simulink model "modelo_i"  (R2026a)
settings: Solver=VariableStepAuto  StopTime=1000  FixedStep=1
values from neighbouring files (symbols this model uses):
  theta = 5    [init.m]
settings Model: Creator=honda  LastModifiedBy=honda

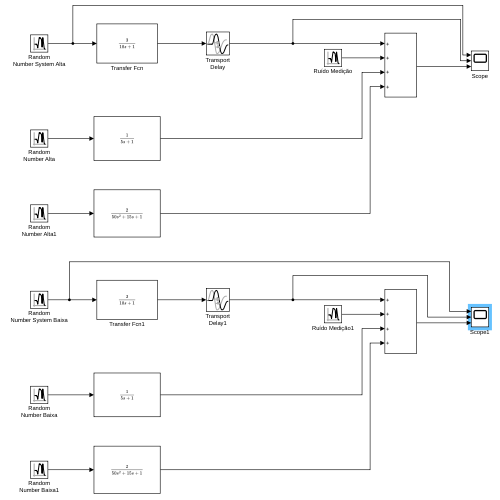
[thumbnail: Simulink's stored preview of the top-level diagram]
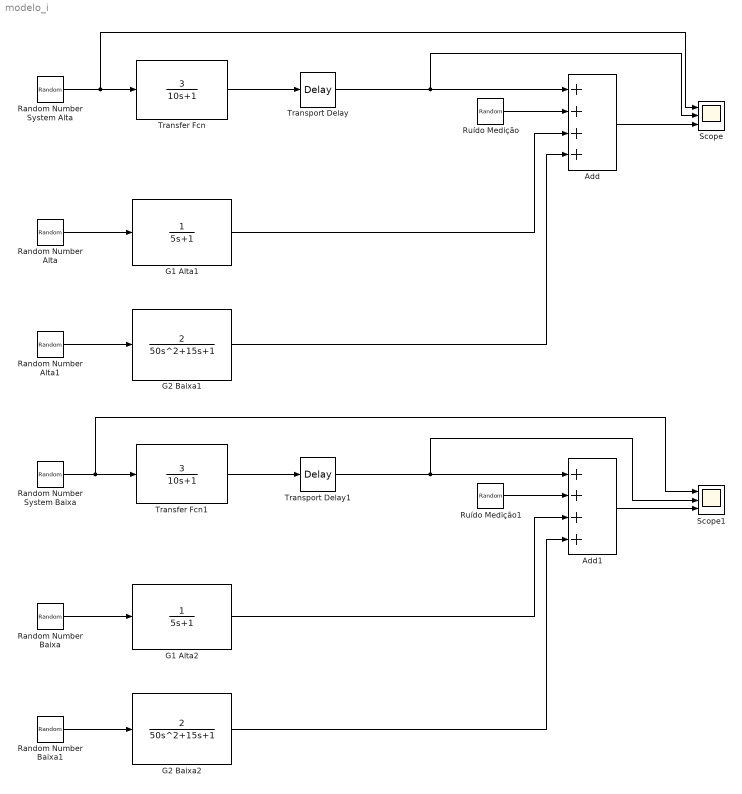
== system modelo_i ==
  Add : Sum  Inputs=++++
  Add1 : Sum  Inputs=++++
  G1 Alta1 : TransferFcn  Denominator=[5 1]
  G1 Alta2 : TransferFcn  Denominator=[5 1]
  G2 Baixa1 : TransferFcn  Numerator=[2]  Denominator=[50 15 1]
  G2 Baixa2 : TransferFcn  Numerator=[2]  Denominator=[50 15 1]
  Random Number Alta : RandomNumber  Variance=0.1  Seed=123  SampleTime=1
  Random Number Alta1 : RandomNumber  Variance=0.1  Seed=456  SampleTime=1
  Random Number Baixa : RandomNumber  Variance=0.001  SampleTime=1
  Random Number Baixa1 : RandomNumber  Variance=0.001  SampleTime=1
  Random Number System Alta : RandomNumber  Variance=0.1  Seed=100  SampleTime=1
  Random Number System Baixa : RandomNumber  Variance=0.1  Seed=100  SampleTime=1
  Ruído Medição : RandomNumber  Variance=1e-6  SampleTime=0.01
  Ruído Medição1 : RandomNumber  Variance=1e-6  SampleTime=0.01
  Scope : Scope  NumInputPorts=3
      settings: ActiveDisplayYMinimum=-1  ActiveDisplayYMaximum=1  DataLoggingVariableName=dados_i_alta
  Scope1 : Scope  NumInputPorts=3
      settings: ActiveDisplayYMinimum=-1  ActiveDisplayYMaximum=1  DataLoggingVariableName=dados_i_baixa
  Transfer Fcn : TransferFcn  Numerator=[3]  Denominator=[10 1]
  Transfer Fcn1 : TransferFcn  Numerator=[3]  Denominator=[10 1]
  Transport Delay : TransportDelay  DelayTime=theta
  Transport Delay1 : TransportDelay  DelayTime=theta
  wires:
  Random Number System Alta/1 -> Scope/1, Transfer Fcn/1
  Transfer Fcn/1 -> Transport Delay/1
  Random Number Alta/1 -> G1 Alta1/1
  Transport Delay/1 -> Scope/2, Add/1
  Ruído Medição/1 -> Add/2
  G1 Alta1/1 -> Add/3
  G2 Baixa1/1 -> Add/4
  Random Number Alta1/1 -> G2 Baixa1/1
  Add/1 -> Scope/3
  G2 Baixa2/1 -> Add1/4
  Transport Delay1/1 -> Scope1/2, Add1/1
  Add1/1 -> Scope1/3
  Random Number System Baixa/1 -> Scope1/1, Transfer Fcn1/1
  Random Number Baixa/1 -> G1 Alta2/1
  Random Number Baixa1/1 -> G2 Baixa2/1
  Transfer Fcn1/1 -> Transport Delay1/1
  G1 Alta2/1 -> Add1/3
  Ruído Medição1/1 -> Add1/2
